simulink model "untitled"  (R2015a)
settings: Solver=ode45  StartTime=0.0  StopTime=10.0  RelTol=1e-3
libraries: cstblocks x12, simulink x12
settings Model: Creator=saadc  LastModifiedBy=saadc

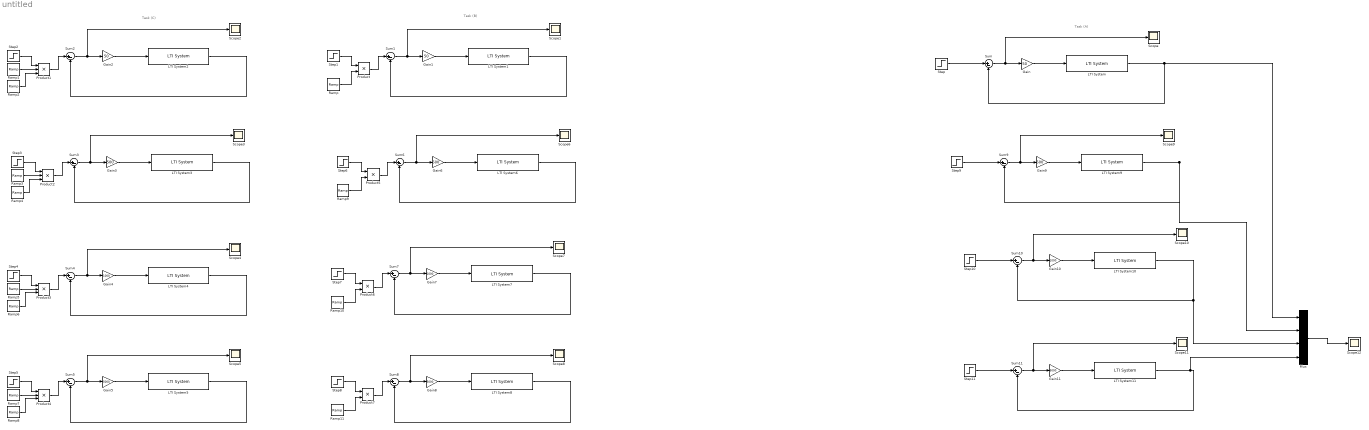
== system untitled ==
  note: Task (C)
  note: Task (B)
  note: Task (A)
  Gain : Gain  Gain=50
  Gain1 : Gain  Gain=50
  Gain10 : Gain  Gain=1000
  Gain11 : Gain  Gain=5000
  Gain2 : Gain  Gain=50
  Gain3 : Gain  Gain=500
  Gain4 : Gain  Gain=1000
  Gain5 : Gain  Gain=5000
  Gain6 : Gain  Gain=500
  Gain7 : Gain  Gain=1000
  Gain8 : Gain  Gain=5000
  Gain9 : Gain  Gain=500
  LTI System{,1..11} (12 alike) : cstblocks/LTI System  sys=tf([1 6],[1 32 367 1776 3024])  IC=[]
  Mux : Mux
  Product{,5..7} (4 alike) : Product
  Product{1..4} (4 alike) : Product  Inputs=3
  Ramp{,1..11} (12 alike) : simulink/Sources/Ramp  slope=1  start=0  X0=0
  Scope{,1..12} (13 alike) : Scope
      Scope settings: YMin=-1  YMax=1
      Scope1 settings: YMin=-1  YMax=1
      Scope10 settings: YMin=-1  YMax=1  SaveName=ScopeData10
      Scope11 settings: YMin=-1  YMax=1  SaveName=ScopeData11
      Scope12 settings: YMin=-1  YMax=1  SaveName=ScopeData12
      Scope2 settings: YMin=-1  YMax=1  SaveName=ScopeData2
      Scope3 settings: YMin=-1  YMax=1  SaveName=ScopeData3
      Scope4 settings: YMin=-1  YMax=1  SaveName=ScopeData4
      Scope5 settings: YMin=-1  YMax=1  SaveName=ScopeData5
      Scope6 settings: YMin=-1  YMax=1  SaveName=ScopeData6
      Scope7 settings: YMin=-1  YMax=1  SaveName=ScopeData7
      Scope8 settings: YMin=-1  YMax=1  SaveName=ScopeData8
      Scope9 settings: YMin=-1  YMax=1  SaveName=ScopeData9
  Step{,1..11} (12 alike) : Step  After=5  SampleTime=0
  Sum{,1..11} (12 alike) : Sum  Inputs=|+-
  wires:
  Step/1 -> Sum/1
  Sum/1 -> Scope/1, Gain/1
  Gain/1 -> LTI System/1
  LTI System/1 -> Mux/1, Sum/2
  Sum1/1 -> Scope1/1, Gain1/1
  Gain1/1 -> LTI System1/1
  LTI System1/1 -> Sum1/2
  Ramp/1 -> Product/2
  Step1/1 -> Product/1
  Product/1 -> Sum1/1
  Sum2/1 -> Scope2/1, Gain2/1
  Gain2/1 -> LTI System2/1
  LTI System2/1 -> Sum2/2
  Ramp1/1 -> Product1/2
  Step2/1 -> Product1/1
  Product1/1 -> Sum2/1
  Ramp2/1 -> Product1/3
  Sum3/1 -> Scope3/1, Gain3/1
  Gain3/1 -> LTI System3/1
  LTI System3/1 -> Sum3/2
  Ramp3/1 -> Product2/2
  Step3/1 -> Product2/1
  Product2/1 -> Sum3/1
  Ramp4/1 -> Product2/3
  Sum4/1 -> Scope4/1, Gain4/1
  Gain4/1 -> LTI System4/1
  LTI System4/1 -> Sum4/2
  Ramp5/1 -> Product3/2
  Step4/1 -> Product3/1
  Product3/1 -> Sum4/1
  Ramp6/1 -> Product3/3
  Sum5/1 -> Scope5/1, Gain5/1
  Gain5/1 -> LTI System5/1
  LTI System5/1 -> Sum5/2
  Ramp7/1 -> Product4/2
  Step5/1 -> Product4/1
  Product4/1 -> Sum5/1
  Ramp8/1 -> Product4/3
  Sum6/1 -> Scope6/1, Gain6/1
  Gain6/1 -> LTI System6/1
  LTI System6/1 -> Sum6/2
  Ramp9/1 -> Product5/2
  Step6/1 -> Product5/1
  Product5/1 -> Sum6/1
  Sum7/1 -> Scope7/1, Gain7/1
  Gain7/1 -> LTI System7/1
  LTI System7/1 -> Sum7/2
  Ramp10/1 -> Product6/2
  Step7/1 -> Product6/1
  Product6/1 -> Sum7/1
  Sum8/1 -> Scope8/1, Gain8/1
  Gain8/1 -> LTI System8/1
  LTI System8/1 -> Sum8/2
  Ramp11/1 -> Product7/2
  Step8/1 -> Product7/1
  Product7/1 -> Sum8/1
  Step9/1 -> Sum9/1
  Sum9/1 -> Scope9/1, Gain9/1
  Gain9/1 -> LTI System9/1
  LTI System9/1 -> Mux/2, Sum9/2
  Step10/1 -> Sum10/1
  Sum10/1 -> Scope10/1, Gain10/1
  Gain10/1 -> LTI System10/1
  LTI System10/1 -> Mux/3, Sum10/2
  Step11/1 -> Sum11/1
  Sum11/1 -> Scope11/1, Gain11/1
  Gain11/1 -> LTI System11/1
  LTI System11/1 -> Mux/4, Sum11/2
  Mux/1 -> Scope12/1
